simulink model "SkywalkerX8_Longitudinal_Control"  (R2018a)
settings: Solver=FixedStepAuto  StartTime=0.0  StopTime=inf  FixedStep=0.02  RelTol=1e-3
undefined symbols (not defined in the file): SkywalkerX8
libraries: simulink x4
settings Model: EnablePacing=on  Creator=David  LastModifiedBy=David

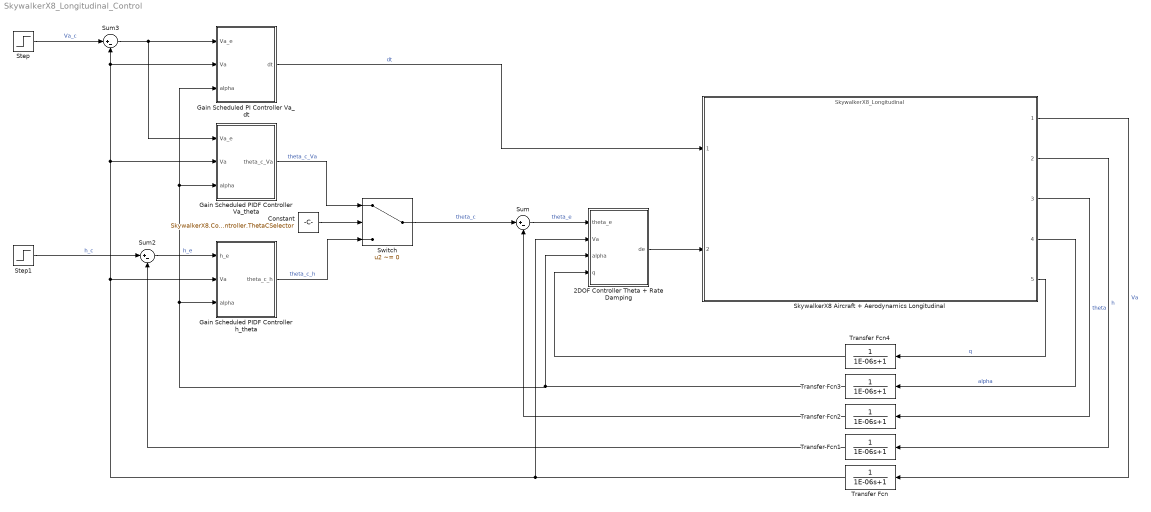
== system SkywalkerX8_Longitudinal_Control ==
  2DOF Controller Theta + Rate Damping : Subsystem
  Constant : Constant  Value=SkywalkerX8.Control.Longitudinal.AlgebraicDesign.ReducedOrderModel.Controller.ThetaCSelector
  Gain Scheduled PI Controller Va_dt : Subsystem
  Gain Scheduled PIDF Controller Va_theta : Subsystem
  Gain Scheduled PIDF Controller h_theta : Subsystem
  SkywalkerX8 Aircraft + Aerodynamics Longitudinal : ModelReference  ModelNameDialog=SkywalkerX8_Longitudinal  ModelReferenceVersion=1.45
      mask Display:
      | image('x8SkySunset.png', 'center')
      | 
      | port_label('input', 1, '\delta_t (Unitless)', 'texmode', 'on')
      | port_label('input', 2, '\delta_e (rad)', 'texmode', 'on')
      | 
      | port_label('output', 1, 'V_a (m/s)', 'texmode', 'on')
      | port_label('output', 2, 'Altitude (m)', 'texmode', 'on')
      | port_label('output', 3, '\theta (rad)', 'texmode', 'on')
      | port_label('output', 4, 'alpha (rad)', 'texmode', 'on')
      | port_label('output', 5, 'q (rad/s)', 'texmode', 'on')
  Step : Step  SampleTime=0
  Step1 : Step  SampleTime=0
  Sum : Sum  Inputs=|+-
  Sum2 : Sum  Inputs=|+-
  Sum3 : Sum  Inputs=|+-
  Switch : Switch  Criteria=u2 ~= 0
  Transfer Fcn{,1..4} (5 alike) : TransferFcn  Denominator=[1E-06 1]
  wires:
  SkywalkerX8 Aircraft + Aerodynamics Longitudinal/3 -> Transfer Fcn2/1  "theta"
  SkywalkerX8 Aircraft + Aerodynamics Longitudinal/1 -> Transfer Fcn/1  "Va"
  SkywalkerX8 Aircraft + Aerodynamics Longitudinal/2 -> Transfer Fcn1/1  "h"
  Switch/1 -> Sum/1  "theta_c"
  Step/1 -> Sum3/1  "Va_c"
  Step1/1 -> Sum2/1  "h_c"
  Gain Scheduled PIDF Controller Va_theta/1(theta_c_Va) -> Switch/1  "theta_c_Va"
  SkywalkerX8 Aircraft + Aerodynamics Longitudinal/5 -> Transfer Fcn4/1  "q"
  Sum3/1 -> Gain Scheduled PI Controller Va_dt/1(Va_e), Gain Scheduled PIDF Controller Va_theta/1(Va_e)
  Gain Scheduled PIDF Controller h_theta/1(theta_c_h) -> Switch/3  "theta_c_h"
  Gain Scheduled PI Controller Va_dt/1(dt) -> SkywalkerX8 Aircraft + Aerodynamics Longitudinal/1  "dt"
  Sum/1 -> 2DOF Controller Theta + Rate Damping/1(theta_e)  "theta_e"
  2DOF Controller Theta + Rate Damping/1(de) -> SkywalkerX8 Aircraft + Aerodynamics Longitudinal/2
  Sum2/1 -> Gain Scheduled PIDF Controller h_theta/1(h_e)  "h_e"
  SkywalkerX8 Aircraft + Aerodynamics Longitudinal/4 -> Transfer Fcn3/1  "alpha"
  Constant/1 -> Switch/2
  Transfer Fcn/1 -> 2DOF Controller Theta + Rate Damping/2(Va), Gain Scheduled PIDF Controller h_theta/2(Va), Gain Scheduled PIDF Controller Va_theta/2(Va), Gain Scheduled PI Controller Va_dt/2(Va), Sum3/2
  Transfer Fcn1/1 -> Sum2/2
  Transfer Fcn2/1 -> Sum/2
  Transfer Fcn3/1 -> Gain Scheduled PIDF Controller h_theta/3(alpha), Gain Scheduled PIDF Controller Va_theta/3(alpha), Gain Scheduled PI Controller Va_dt/3(alpha), 2DOF Controller Theta + Rate Damping/3(alpha)
  Transfer Fcn4/1 -> 2DOF Controller Theta + Rate Damping/4(q)

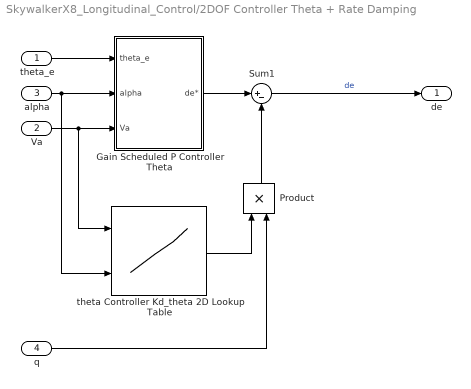
== system SkywalkerX8_Longitudinal_Control/2DOF Controller Theta + Rate Damping ==
  theta_e : Inport
  Va : Inport  Port=2
  alpha : Inport  Port=3
  q : Inport  Port=4
  Gain Scheduled P Controller Theta : Subsystem
  Product : Product
  Sum1 : Sum  Inputs=|+-
  theta Controller Kd_theta 2D Lookup Table : Lookup_n-D  BreakpointsForDimension1=[1 2 3 4 5]  BreakpointsForDimension2=[1 2 3 4 5]  Table=ones(5, 5)  InternalRulePriority=Speed  RndMeth=Simplest  InputSameDT=on
  de : Outport
  wires:
  Gain Scheduled P Controller Theta/1(de*) -> Sum1/1
  alpha/1 -> theta Controller Kd_theta 2D Lookup Table/2, Gain Scheduled P Controller Theta/2(alpha)
  Sum1/1 -> de/1  "de"
  theta_e/1 -> Gain Scheduled P Controller Theta/1(theta_e)
  Va/1 -> theta Controller Kd_theta 2D Lookup Table/1, Gain Scheduled P Controller Theta/3(Va)
  q/1 -> Product/2
  theta Controller Kd_theta 2D Lookup Table/1 -> Product/1
  Product/1 -> Sum1/2

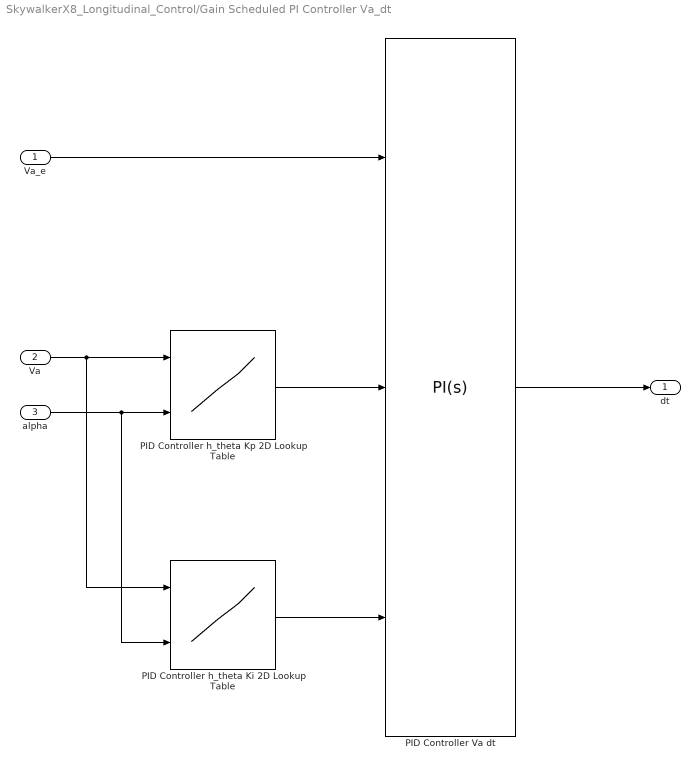
== system SkywalkerX8_Longitudinal_Control/Gain Scheduled PI Controller Va_dt ==
  Va_e : Inport
  Va : Inport  Port=2
  alpha : Inport  Port=3
  PID Controller Va dt : simulink/Continuous/PID Controller  Controller=PI  TimeDomain=Continuous-time  SampleTime=-1  IntegratorMethod=Forward Euler  FilterMethod=Forward Euler  Form=Parallel  UseFilter=on  ControllerParametersSource=external  P=-0.520426076441774  I=-5.25943351691776e-08  D=0  N=100  InitialConditionSource=internal  InitialConditionForIntegrator=0  InitialConditionForFilter=0  ExternalReset=none  IgnoreLimit=on  LimitOutput=off  UpperSaturationLimit=1  LowerSaturationLimit=0  LinearizeAsGain=on  AntiWindupMode=clamping  Kb=1  TrackingMode=off  Kt=1  PParamMin=[]  PParamMax=[]  IParamMin=[]  IParamMax=[]  DParamMin=[]  DParamMax=[]  NParamMin=[]  NParamMax=[]  KbParamMin=[]  KbParamMax=[]  KtParamMin=[]  KtParamMax=[]  POutMin=[]  POutMax=[]  IOutMin=[]  IOutMax=[]  DOutMin=[]  DOutMax=[]  NOutMin=[]  NOutMax=[]  KbOutMin=[]  KbOutMax=[]  KtOutMin=[]  KtOutMax=[]  IntegratorOutMin=[]  IntegratorOutMax=[]  FilterOutMin=[]  FilterOutMax=[]  SumOutMin=[]  SumOutMax=[]  SumI1OutMin=[]  SumI1OutMax=[]  SumI2OutMin=[]  SumI2OutMax=[]  SumI3OutMin=[]  SumI3OutMax=[]  SumDOutMin=[]  SumDOutMax=[]  SaturationOutMin=[]  SaturationOutMax=[]  IntegratorContinuousStateAttributes=''  IntegratorStateMustResolveToSignalObject=off  IntegratorRTWStateStorageClass=Auto  FilterContinuousStateAttributes=''  FilterStateMustResolveToSignalObject=off  FilterRTWStateStorageClass=Auto  DifferentiatorICPrevScaledInput=0  DifferentiatorOutMin=[]  DifferentiatorOutMax=[]  FilterDiffOutCoefMin=[]  FilterDiffOutCoefMax=[]  SumDenOutMin=[]  SumDenOutMax=[]  SumNumOutMin=[]  SumNumOutMax=[]  ReciprocalOutMin=[]  ReciprocalOutMax=[]  DivideOutMin=[]  DivideOutMax=[]  TunerSelectOption=Transfer Function Based (PID Tuner App)
  PID Controller h_theta Ki 2D Lookup Table : Lookup_n-D  BreakpointsForDimension1=[1 2 3 4 5]  BreakpointsForDimension2=[1 2 3 4 5]  Table=ones(5, 5)  InternalRulePriority=Speed  RndMeth=Simplest  InputSameDT=on
  PID Controller h_theta Kp 2D Lookup Table : Lookup_n-D  BreakpointsForDimension1=[1 2 3 4 5]  BreakpointsForDimension2=[1 2 3 4 5]  Table=ones(5, 5)  InternalRulePriority=Speed  RndMeth=Simplest  InputSameDT=on
  dt : Outport
  wires:
  Va_e/1 -> PID Controller Va dt/1
  PID Controller Va dt/1 -> dt/1
  PID Controller h_theta Kp 2D Lookup Table/1 -> PID Controller Va dt/2
  Va/1 -> PID Controller h_theta Ki 2D Lookup Table/1, PID Controller h_theta Kp 2D Lookup Table/1
  PID Controller h_theta Ki 2D Lookup Table/1 -> PID Controller Va dt/3
  alpha/1 -> PID Controller h_theta Ki 2D Lookup Table/2, PID Controller h_theta Kp 2D Lookup Table/2

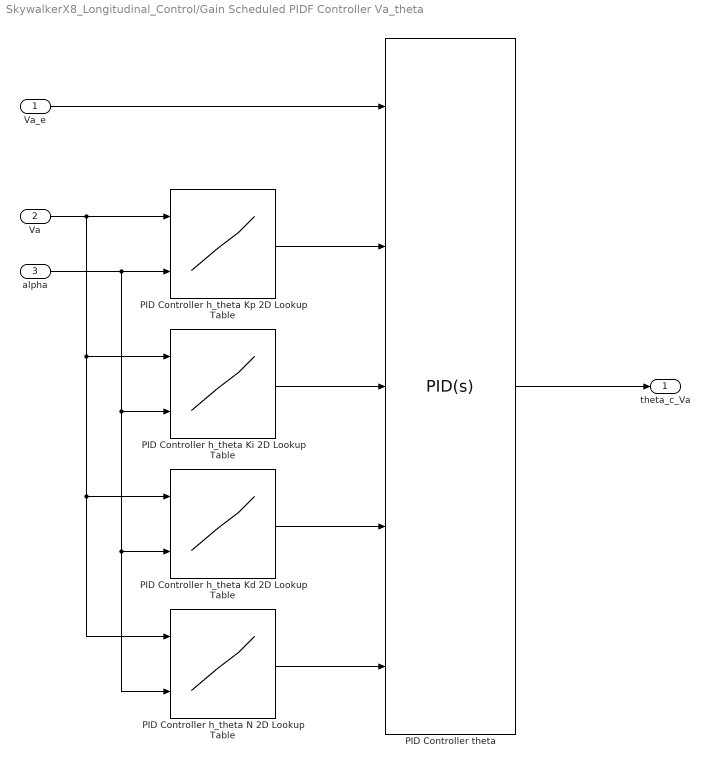
== system SkywalkerX8_Longitudinal_Control/Gain Scheduled PIDF Controller Va_theta ==
  Va_e : Inport
  Va : Inport  Port=2
  alpha : Inport  Port=3
  PID Controller h_theta Kd 2D Lookup Table : Lookup_n-D  BreakpointsForDimension1=[1:3]  BreakpointsForDimension2=[1:3]  InternalRulePriority=Speed  RndMeth=Simplest  InputSameDT=on
  PID Controller h_theta Ki 2D Lookup Table : Lookup_n-D  BreakpointsForDimension1=[1:3]  BreakpointsForDimension2=[1:3]  InternalRulePriority=Speed  RndMeth=Simplest  InputSameDT=on
  PID Controller h_theta Kp 2D Lookup Table : Lookup_n-D  BreakpointsForDimension1=[1:3]  BreakpointsForDimension2=[1:3]  InternalRulePriority=Speed  RndMeth=Simplest  InputSameDT=on
  PID Controller h_theta N 2D Lookup Table : Lookup_n-D  BreakpointsForDimension1=[1:3]  BreakpointsForDimension2=[1:3]  InternalRulePriority=Speed  RndMeth=Simplest  InputSameDT=on
  PID Controller theta : simulink/Continuous/PID Controller  Controller=PID  TimeDomain=Continuous-time  SampleTime=-1  IntegratorMethod=Forward Euler  FilterMethod=Forward Euler  Form=Parallel  UseFilter=on  ControllerParametersSource=external  P=-0.520426076441774  I=-5.25943351691776e-08  D=0  N=100  InitialConditionSource=internal  InitialConditionForIntegrator=0  InitialConditionForFilter=0  ExternalReset=none  IgnoreLimit=on  LimitOutput=on  UpperSaturationLimit=15*pi/180  LowerSaturationLimit=-15*pi/180  LinearizeAsGain=on  AntiWindupMode=clamping  Kb=1  TrackingMode=off  Kt=1  PParamMin=[]  PParamMax=[]  IParamMin=[]  IParamMax=[]  DParamMin=[]  DParamMax=[]  NParamMin=[]  NParamMax=[]  KbParamMin=[]  KbParamMax=[]  KtParamMin=[]  KtParamMax=[]  POutMin=[]  POutMax=[]  IOutMin=[]  IOutMax=[]  DOutMin=[]  DOutMax=[]  NOutMin=[]  NOutMax=[]  KbOutMin=[]  KbOutMax=[]  KtOutMin=[]  KtOutMax=[]  IntegratorOutMin=[]  IntegratorOutMax=[]  FilterOutMin=[]  FilterOutMax=[]  SumOutMin=[]  SumOutMax=[]  SumI1OutMin=[]  SumI1OutMax=[]  SumI2OutMin=[]  SumI2OutMax=[]  SumI3OutMin=[]  SumI3OutMax=[]  SumDOutMin=[]  SumDOutMax=[]  SaturationOutMin=[]  SaturationOutMax=[]  IntegratorContinuousStateAttributes=''  IntegratorStateMustResolveToSignalObject=off  IntegratorRTWStateStorageClass=Auto  FilterContinuousStateAttributes=''  FilterStateMustResolveToSignalObject=off  FilterRTWStateStorageClass=Auto  DifferentiatorICPrevScaledInput=0  DifferentiatorOutMin=[]  DifferentiatorOutMax=[]  FilterDiffOutCoefMin=[]  FilterDiffOutCoefMax=[]  SumDenOutMin=[]  SumDenOutMax=[]  SumNumOutMin=[]  SumNumOutMax=[]  ReciprocalOutMin=[]  ReciprocalOutMax=[]  DivideOutMin=[]  DivideOutMax=[]  TunerSelectOption=Transfer Function Based (PID Tuner App)
  theta_c_Va : Outport
  wires:
  Va_e/1 -> PID Controller theta/1
  PID Controller theta/1 -> theta_c_Va/1
  PID Controller h_theta Kp 2D Lookup Table/1 -> PID Controller theta/2
  Va/1 -> PID Controller h_theta Kd 2D Lookup Table/1, PID Controller h_theta N 2D Lookup Table/1, PID Controller h_theta Ki 2D Lookup Table/1, PID Controller h_theta Kp 2D Lookup Table/1
  PID Controller h_theta Ki 2D Lookup Table/1 -> PID Controller theta/3
  PID Controller h_theta Kd 2D Lookup Table/1 -> PID Controller theta/4
  PID Controller h_theta N 2D Lookup Table/1 -> PID Controller theta/5
  alpha/1 -> PID Controller h_theta N 2D Lookup Table/2, PID Controller h_theta Kd 2D Lookup Table/2, PID Controller h_theta Ki 2D Lookup Table/2, PID Controller h_theta Kp 2D Lookup Table/2

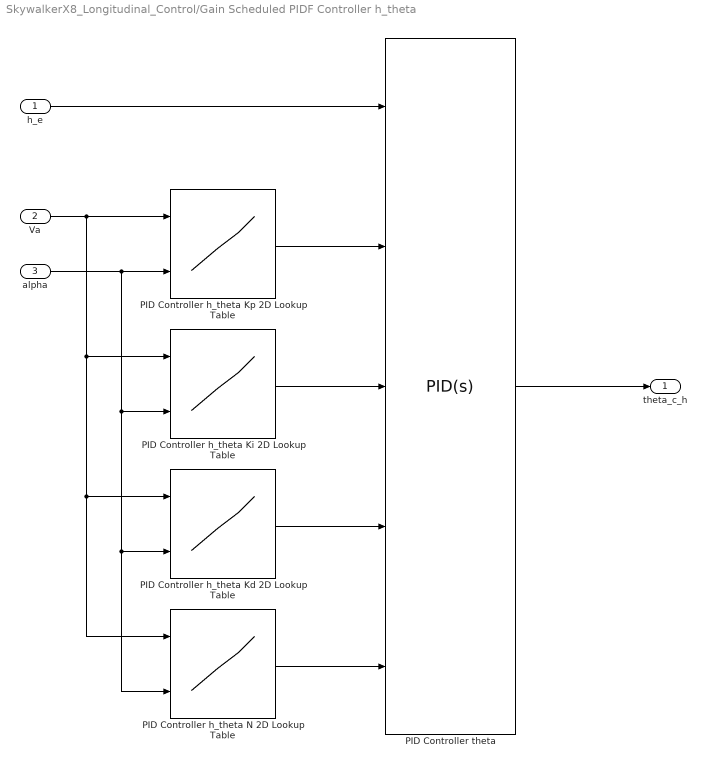
== system SkywalkerX8_Longitudinal_Control/Gain Scheduled PIDF Controller h_theta ==
  h_e : Inport
  Va : Inport  Port=2
  alpha : Inport  Port=3
  PID Controller h_theta Kd 2D Lookup Table : Lookup_n-D  BreakpointsForDimension1=[1:3]  BreakpointsForDimension2=[1:3]  InternalRulePriority=Speed  RndMeth=Simplest  InputSameDT=on
  PID Controller h_theta Ki 2D Lookup Table : Lookup_n-D  BreakpointsForDimension1=[1:3]  BreakpointsForDimension2=[1:3]  InternalRulePriority=Speed  RndMeth=Simplest  InputSameDT=on
  PID Controller h_theta Kp 2D Lookup Table : Lookup_n-D  BreakpointsForDimension1=[1:3]  BreakpointsForDimension2=[1:3]  InternalRulePriority=Speed  RndMeth=Simplest  InputSameDT=on
  PID Controller h_theta N 2D Lookup Table : Lookup_n-D  BreakpointsForDimension1=[1:3]  BreakpointsForDimension2=[1:3]  InternalRulePriority=Speed  RndMeth=Simplest  InputSameDT=on
  PID Controller theta : simulink/Continuous/PID Controller  Controller=PID  TimeDomain=Continuous-time  SampleTime=-1  IntegratorMethod=Forward Euler  FilterMethod=Forward Euler  Form=Parallel  UseFilter=on  ControllerParametersSource=external  P=-0.520426076441774  I=-5.25943351691776e-08  D=0  N=100  InitialConditionSource=internal  InitialConditionForIntegrator=0  InitialConditionForFilter=0  ExternalReset=none  IgnoreLimit=on  LimitOutput=off  UpperSaturationLimit=15*pi/180  LowerSaturationLimit=-15*pi/180  LinearizeAsGain=on  AntiWindupMode=clamping  Kb=1  TrackingMode=off  Kt=1  PParamMin=[]  PParamMax=[]  IParamMin=[]  IParamMax=[]  DParamMin=[]  DParamMax=[]  NParamMin=[]  NParamMax=[]  KbParamMin=[]  KbParamMax=[]  KtParamMin=[]  KtParamMax=[]  POutMin=[]  POutMax=[]  IOutMin=[]  IOutMax=[]  DOutMin=[]  DOutMax=[]  NOutMin=[]  NOutMax=[]  KbOutMin=[]  KbOutMax=[]  KtOutMin=[]  KtOutMax=[]  IntegratorOutMin=[]  IntegratorOutMax=[]  FilterOutMin=[]  FilterOutMax=[]  SumOutMin=[]  SumOutMax=[]  SumI1OutMin=[]  SumI1OutMax=[]  SumI2OutMin=[]  SumI2OutMax=[]  SumI3OutMin=[]  SumI3OutMax=[]  SumDOutMin=[]  SumDOutMax=[]  SaturationOutMin=[]  SaturationOutMax=[]  IntegratorContinuousStateAttributes=''  IntegratorStateMustResolveToSignalObject=off  IntegratorRTWStateStorageClass=Auto  FilterContinuousStateAttributes=''  FilterStateMustResolveToSignalObject=off  FilterRTWStateStorageClass=Auto  DifferentiatorICPrevScaledInput=0  DifferentiatorOutMin=[]  DifferentiatorOutMax=[]  FilterDiffOutCoefMin=[]  FilterDiffOutCoefMax=[]  SumDenOutMin=[]  SumDenOutMax=[]  SumNumOutMin=[]  SumNumOutMax=[]  ReciprocalOutMin=[]  ReciprocalOutMax=[]  DivideOutMin=[]  DivideOutMax=[]  TunerSelectOption=Transfer Function Based (PID Tuner App)
  theta_c_h : Outport
  wires:
  h_e/1 -> PID Controller theta/1
  PID Controller theta/1 -> theta_c_h/1
  PID Controller h_theta Kp 2D Lookup Table/1 -> PID Controller theta/2
  Va/1 -> PID Controller h_theta Kd 2D Lookup Table/1, PID Controller h_theta N 2D Lookup Table/1, PID Controller h_theta Ki 2D Lookup Table/1, PID Controller h_theta Kp 2D Lookup Table/1
  PID Controller h_theta Ki 2D Lookup Table/1 -> PID Controller theta/3
  PID Controller h_theta Kd 2D Lookup Table/1 -> PID Controller theta/4
  PID Controller h_theta N 2D Lookup Table/1 -> PID Controller theta/5
  alpha/1 -> PID Controller h_theta N 2D Lookup Table/2, PID Controller h_theta Kd 2D Lookup Table/2, PID Controller h_theta Ki 2D Lookup Table/2, PID Controller h_theta Kp 2D Lookup Table/2

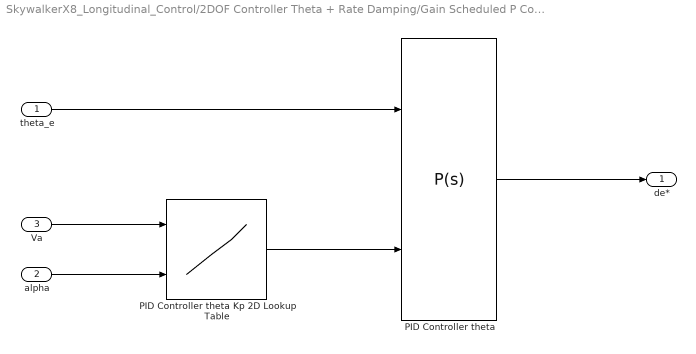
== system SkywalkerX8_Longitudinal_Control/2DOF Controller Theta + Rate Damping/Gain Scheduled P Controller Theta ==
  theta_e : Inport
  alpha : Inport  Port=2
  Va : Inport  Port=3
  PID Controller theta : simulink/Continuous/PID Controller  Controller=P  TimeDomain=Continuous-time  SampleTime=-1  IntegratorMethod=Forward Euler  FilterMethod=Forward Euler  Form=Parallel  UseFilter=on  ControllerParametersSource=external  P=-0.520426076441774  I=-5.25943351691776e-08  D=0  N=100  InitialConditionSource=internal  InitialConditionForIntegrator=0  InitialConditionForFilter=0  ExternalReset=none  IgnoreLimit=on  LimitOutput=off  UpperSaturationLimit=15*pi/180  LowerSaturationLimit=-15*pi/180  LinearizeAsGain=on  AntiWindupMode=clamping  Kb=1  TrackingMode=off  Kt=1  PParamMin=[]  PParamMax=[]  IParamMin=[]  IParamMax=[]  DParamMin=[]  DParamMax=[]  NParamMin=[]  NParamMax=[]  KbParamMin=[]  KbParamMax=[]  KtParamMin=[]  KtParamMax=[]  POutMin=[]  POutMax=[]  IOutMin=[]  IOutMax=[]  DOutMin=[]  DOutMax=[]  NOutMin=[]  NOutMax=[]  KbOutMin=[]  KbOutMax=[]  KtOutMin=[]  KtOutMax=[]  IntegratorOutMin=[]  IntegratorOutMax=[]  FilterOutMin=[]  FilterOutMax=[]  SumOutMin=[]  SumOutMax=[]  SumI1OutMin=[]  SumI1OutMax=[]  SumI2OutMin=[]  SumI2OutMax=[]  SumI3OutMin=[]  SumI3OutMax=[]  SumDOutMin=[]  SumDOutMax=[]  SaturationOutMin=[]  SaturationOutMax=[]  IntegratorContinuousStateAttributes=''  IntegratorStateMustResolveToSignalObject=off  IntegratorRTWStateStorageClass=Auto  FilterContinuousStateAttributes=''  FilterStateMustResolveToSignalObject=off  FilterRTWStateStorageClass=Auto  DifferentiatorICPrevScaledInput=0  DifferentiatorOutMin=[]  DifferentiatorOutMax=[]  FilterDiffOutCoefMin=[]  FilterDiffOutCoefMax=[]  SumDenOutMin=[]  SumDenOutMax=[]  SumNumOutMin=[]  SumNumOutMax=[]  ReciprocalOutMin=[]  ReciprocalOutMax=[]  DivideOutMin=[]  DivideOutMax=[]  TunerSelectOption=Transfer Function Based (PID Tuner App)
  PID Controller theta Kp 2D Lookup Table : Lookup_n-D  BreakpointsForDimension1=[1 2 3 4 5]  BreakpointsForDimension2=[1 2 3 4 5]  Table=ones(5, 5)  InternalRulePriority=Speed  RndMeth=Simplest  InputSameDT=on
  de* : Outport
  wires:
  theta_e/1 -> PID Controller theta/1
  PID Controller theta/1 -> de*/1
  PID Controller theta Kp 2D Lookup Table/1 -> PID Controller theta/2
  alpha/1 -> PID Controller theta Kp 2D Lookup Table/2
  Va/1 -> PID Controller theta Kp 2D Lookup Table/1
